simulink model "punto3_simulink_parte2"  (R2024a)
settings: Solver=VariableStepAuto  StartTime=0.0  StopTime=20  RelTol=1e-3
undefined symbols (not defined in the file): A, B, C, D
libraries: fuzblock x2
settings Model: Creator=USER  LastModifiedBy=USER

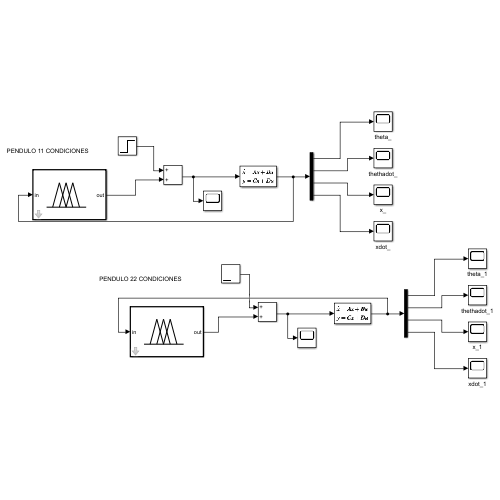
[thumbnail: Simulink's stored preview of the top-level diagram]
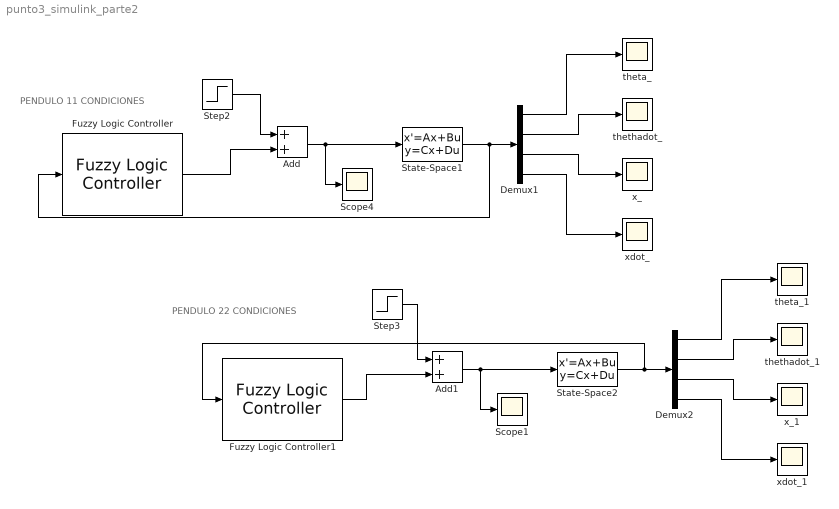
== system punto3_simulink_parte2 ==
  note: PENDULO 11 CONDICIONES
  note: PENDULO 22 CONDICIONES
  Add : Sum
  Add1 : Sum
  Demux1 : Demux
  Demux2 : Demux
  Fuzzy Logic Controller : fuzblock/Fuzzy Logic  Controller  FIS='pendulo.fis'  OutputSampleNumber=101  DataType=double  FuzzifiedInputs=off  RuleFiringStrengths=off  RuleOutputs=off  AggregatedOutputs=off  SimulateUsing=Code generation  OutOfRangeInputValueMessage=warning  NoRuleFiredMessage=warning  EmptyOutputFuzzySetMessage=warning
  Fuzzy Logic Controller1 : fuzblock/Fuzzy Logic  Controller  FIS='pendulo2.fis'  OutputSampleNumber=101  DataType=double  FuzzifiedInputs=off  RuleFiringStrengths=off  RuleOutputs=off  AggregatedOutputs=off  SimulateUsing=Code generation  OutOfRangeInputValueMessage=warning  NoRuleFiredMessage=warning  EmptyOutputFuzzySetMessage=warning
  Scope1 : Scope
  Scope4 : Scope
  State-Space1 : StateSpace  A=A  B=B  C=C  D=D  InitialCondition=0
  State-Space2 : StateSpace  A=A  B=B  C=C  D=D  InitialCondition=0
  Step2 : Step  Time=2  Before=10  After=10  SampleTime=0
  Step3 : Step  Time=2  Before=10  After=10  SampleTime=0
  theta_ : Scope
  theta_1 : Scope
  thethadot_ : Scope
  thethadot_1 : Scope
  x_ : Scope
  x_1 : Scope
  xdot_ : Scope
  xdot_1 : Scope
  wires:
  Demux1/2 -> thethadot_/1
  Add/1 -> State-Space1/1, Scope4/1
  State-Space1/1 -> Fuzzy Logic Controller/1, Demux1/1
  Demux1/4 -> xdot_/1
  Fuzzy Logic Controller/1 -> Add/2
  Demux1/3 -> x_/1
  Demux1/1 -> theta_/1
  Step2/1 -> Add/1
  Fuzzy Logic Controller1/1 -> Add1/2
  Step3/1 -> Add1/1
  Demux2/3 -> x_1/1
  Demux2/4 -> xdot_1/1
  Demux2/1 -> theta_1/1
  State-Space2/1 -> Fuzzy Logic Controller1/1, Demux2/1
  Demux2/2 -> thethadot_1/1
  Add1/1 -> State-Space2/1, Scope1/1
